simulink model "tx2"  (R2022a)
settings: Solver=FixedStepDiscrete  StartTime=0.0  StopTime=3.1e6  FixedStep=1  RelTol=1e-3
undefined symbols (not defined in the file or in its folder): rom_bf1, rom_bf2, rom_bf3, rom_bf4, rom_bf5, rom_bf6, rom_bf7, rom_bf8, rom_pilot_tt
libraries: hdlsllib x809, whdlutilities x460, whdlmod x104, whdledac x26, simulink x3
(part 4 of 27)

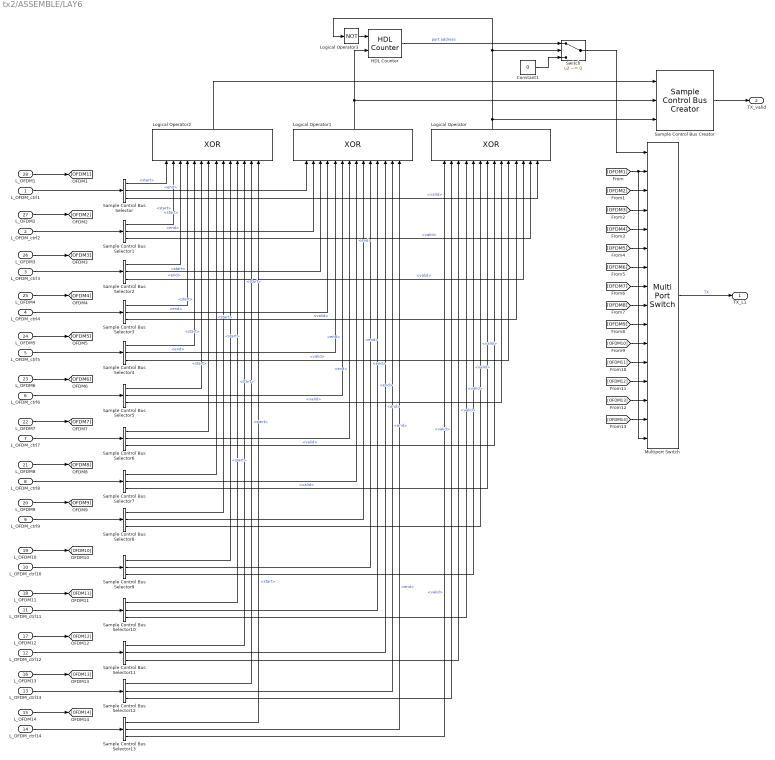
== system tx2/ASSEMBLE/LAY6 ==
  L_OFDM_ctrl1 : Inport  OutDataTypeStr=Bus: samplecontrol
  L_OFDM_ctrl2 : Inport  Port=2  OutDataTypeStr=Bus: samplecontrol
  L_OFDM_ctrl3 : Inport  Port=3  OutDataTypeStr=Bus: samplecontrol
  L_OFDM_ctrl4 : Inport  Port=4  OutDataTypeStr=Bus: samplecontrol
  L_OFDM_ctrl5 : Inport  Port=5  OutDataTypeStr=Bus: samplecontrol
  L_OFDM_ctrl6 : Inport  Port=6  OutDataTypeStr=Bus: samplecontrol
  L_OFDM_ctrl7 : Inport  Port=7  OutDataTypeStr=Bus: samplecontrol
  L_OFDM_ctrl8 : Inport  Port=8  OutDataTypeStr=Bus: samplecontrol
  L_OFDM_ctrl9 : Inport  Port=9  OutDataTypeStr=Bus: samplecontrol
  L_OFDM_ctrl10 : Inport  Port=10  OutDataTypeStr=Bus: samplecontrol
  L_OFDM_ctrl11 : Inport  Port=11  OutDataTypeStr=Bus: samplecontrol
  L_OFDM_ctrl12 : Inport  Port=12  OutDataTypeStr=Bus: samplecontrol
  L_OFDM_ctrl13 : Inport  Port=13  OutDataTypeStr=Bus: samplecontrol
  L_OFDM_ctrl14 : Inport  Port=14  OutDataTypeStr=Bus: samplecontrol
  L_OFDM14 : Inport  Port=15
  L_OFDM13 : Inport  Port=16
  L_OFDM12 : Inport  Port=17
  L_OFDM11 : Inport  Port=18
  L_OFDM10 : Inport  Port=19
  L_OFDM9 : Inport  Port=20
  L_OFDM8 : Inport  Port=21
  L_OFDM7 : Inport  Port=22
  L_OFDM6 : Inport  Port=23
  L_OFDM5 : Inport  Port=24
  L_OFDM4 : Inport  Port=25
  L_OFDM3 : Inport  Port=26
  L_OFDM2 : Inport  Port=27
  L_OFDM1 : Inport  Port=28
  Constant1 : Constant  Value=0  OutDataTypeStr=uint8
  HDL Counter : hdlsllib/Sources/HDL Counter  CountType=Count limited  CountInit=0  CountStep=1  CountMax=13  CountFromType=Initial value  CountFrom=0  CountResetPort=on  CountLoadPort=off  CountEnbPort=on  CountDirPort=off  CountHitOutputPort=off  CountDataType=Unsigned  CountWordLen=8  CountFracLen=0  CountSampTime=1
  Logical Operator : Logic  Operator=XOR  Inputs=14  AllPortsSameDT=off  OutDataTypeStr=boolean
  Logical Operator1 : Logic  Operator=XOR  Inputs=14  AllPortsSameDT=off  OutDataTypeStr=boolean
  Logical Operator2 : Logic  Operator=XOR  Inputs=14  AllPortsSameDT=off  OutDataTypeStr=boolean
  Logical Operator3 : Logic  Operator=NOT  AllPortsSameDT=off  OutDataTypeStr=boolean
  Multiport Switch : MultiPortSwitch  DataPortOrder=Zero-based contiguous  Inputs=14  DataPortForDefault=Additional data port  zeroidx=on  SaturateOnIntegerOverflow=off  InputSameDT=off
  Sample Control Bus Creator : whdlutilities/Sample Control Bus Creator
      settings: SourceProductBaseCode=LH
  Sample Control Bus Selector{,1..13} (14 alike) : whdlutilities/Sample Control Bus Selector  OutputSignals=start,end,valid
      settings: SourceProductBaseCode=LH
  Switch : Switch  Criteria=u2 ~= 0  SaturateOnIntegerOverflow=off  InputSameDT=off
  TX_L1 : Outport
  TX_valid : Outport  Port=2  OutDataTypeStr=Bus: samplecontrol
  wires:
  Logical Operator2/1 -> Sample Control Bus Creator/1
  Sample Control Bus Creator/1 -> TX_valid/1
  Sample Control Bus Selector13/1 -> Logical Operator2/14  "<start>"
  Sample Control Bus Selector12/1 -> Logical Operator2/13  "<start>"
  Sample Control Bus Selector11/1 -> Logical Operator2/12  "<start>"
  Sample Control Bus Selector10/1 -> Logical Operator2/11  "<start>"
  Sample Control Bus Selector9/1 -> Logical Operator2/10  "<start>"
  Sample Control Bus Selector8/1 -> Logical Operator2/9  "<start>"
  Sample Control Bus Selector7/1 -> Logical Operator2/8  "<start>"
  Sample Control Bus Selector6/1 -> Logical Operator2/7  "<start>"
  Sample Control Bus Selector5/1 -> Logical Operator2/6  "<start>"
  Sample Control Bus Selector4/1 -> Logical Operator2/5  "<start>"
  Sample Control Bus Selector3/1 -> Logical Operator2/4  "<start>"
  Sample Control Bus Selector2/1 -> Logical Operator2/3  "<start>"
  Sample Control Bus Selector1/1 -> Logical Operator2/2  "<start>"
  Sample Control Bus Selector/1 -> Logical Operator2/1  "<start>"
  Multiport Switch/1 -> TX_L1/1  "TX"
  L_OFDM_ctrl11/1 -> Sample Control Bus Selector10/1
  L_OFDM9/1 -> [OFDM9]
  L_OFDM_ctrl1/1 -> Sample Control Bus Selector/1
  L_OFDM_ctrl7/1 -> Sample Control Bus Selector6/1
  L_OFDM_ctrl4/1 -> Sample Control Bus Selector3/1
  L_OFDM_ctrl14/1 -> Sample Control Bus Selector13/1
  L_OFDM_ctrl9/1 -> Sample Control Bus Selector8/1
  L_OFDM_ctrl3/1 -> Sample Control Bus Selector2/1
  L_OFDM7/1 -> [OFDM7]
  L_OFDM6/1 -> [OFDM6]
  L_OFDM14/1 -> [OFDM14]
  L_OFDM_ctrl2/1 -> Sample Control Bus Selector1/1
  L_OFDM_ctrl13/1 -> Sample Control Bus Selector12/1
  Sample Control Bus Selector9/3 -> Logical Operator/5  "<valid>"
  Sample Control Bus Selector9/2 -> Logical Operator1/10  "<end>"
  L_OFDM_ctrl5/1 -> Sample Control Bus Selector4/1
  Sample Control Bus Selector7/2 -> Logical Operator1/8  "<end>"
  L_OFDM_ctrl12/1 -> Sample Control Bus Selector11/1
  [OFDM8] -> Multiport Switch/9
  Sample Control Bus Selector1/2 -> Logical Operator1/2  "<end>"
  Sample Control Bus Selector3/2 -> Logical Operator1/4  "<end>"
  Sample Control Bus Selector13/3 -> Logical Operator/1  "<valid>"
  Sample Control Bus Selector3/3 -> Logical Operator/11  "<valid>"
  [OFDM3] -> Multiport Switch/4
  Sample Control Bus Selector4/2 -> Logical Operator1/5  "<end>"
  Sample Control Bus Selector11/3 -> Logical Operator/3  "<valid>"
  [OFDM11] -> Multiport Switch/12
  L_OFDM4/1 -> [OFDM4]
  Sample Control Bus Selector11/2 -> Logical Operator1/12  "<end>"
  Sample Control Bus Selector4/3 -> Logical Operator/10  "<valid>"
  [OFDM12] -> Multiport Switch/13
  Sample Control Bus Selector2/2 -> Logical Operator1/3  "<end>"
  L_OFDM1/1 -> [OFDM1]
  Constant1/1 -> Switch/3
  L_OFDM11/1 -> [OFDM11]
  L_OFDM12/1 -> [OFDM12]
  Sample Control Bus Selector/2 -> Logical Operator1/1  "<end>"
  Sample Control Bus Selector5/3 -> Logical Operator/9  "<valid>"
  Switch/1 -> Multiport Switch/1
  Sample Control Bus Selector2/3 -> Logical Operator/12  "<valid>"
  [OFDM13] -> Multiport Switch/14
  [OFDM4] -> Multiport Switch/5
  [OFDM5] -> Multiport Switch/6
  HDL Counter/1 -> Switch/1  "port address"
  L_OFDM13/1 -> [OFDM13]
  [OFDM10] -> Multiport Switch/11
  Sample Control Bus Selector8/2 -> Logical Operator1/9  "<end>"
  Sample Control Bus Selector7/3 -> Logical Operator/7  "<valid>"
  L_OFDM_ctrl10/1 -> Sample Control Bus Selector9/1
  L_OFDM_ctrl6/1 -> Sample Control Bus Selector5/1
  [OFDM1] -> Multiport Switch/16, Multiport Switch/2
  Sample Control Bus Selector12/2 -> Logical Operator1/13  "<end>"
  Sample Control Bus Selector13/2 -> Logical Operator1/14  "<end>"
  L_OFDM10/1 -> [OFDM10]
  Sample Control Bus Selector6/2 -> Logical Operator1/7  "<end>"
  [OFDM7] -> Multiport Switch/8
  [OFDM6] -> Multiport Switch/7
  Logical Operator/1 -> Sample Control Bus Creator/3, Switch/2, Logical Operator3/1
  Sample Control Bus Selector6/3 -> Logical Operator/8  "<valid>"
  Sample Control Bus Selector5/2 -> Logical Operator1/6  "<end>"
  [OFDM9] -> Multiport Switch/10
  [OFDM2] -> Multiport Switch/3
  L_OFDM2/1 -> [OFDM2]
  Sample Control Bus Selector12/3 -> Logical Operator/2  "<valid>"
  L_OFDM3/1 -> [OFDM3]
  Sample Control Bus Selector1/3 -> Logical Operator/13  "<valid>"
  L_OFDM8/1 -> [OFDM8]
  Sample Control Bus Selector10/2 -> Logical Operator1/11  "<end>"
  Sample Control Bus Selector/3 -> Logical Operator/14  "<valid>"
  L_OFDM5/1 -> [OFDM5]
  Logical Operator1/1 -> Sample Control Bus Creator/2, HDL Counter/2
  [OFDM14] -> Multiport Switch/15
  Sample Control Bus Selector10/3 -> Logical Operator/4  "<valid>"
  L_OFDM_ctrl8/1 -> Sample Control Bus Selector7/1
  Sample Control Bus Selector8/3 -> Logical Operator/6  "<valid>"
  Logical Operator3/1 -> HDL Counter/1

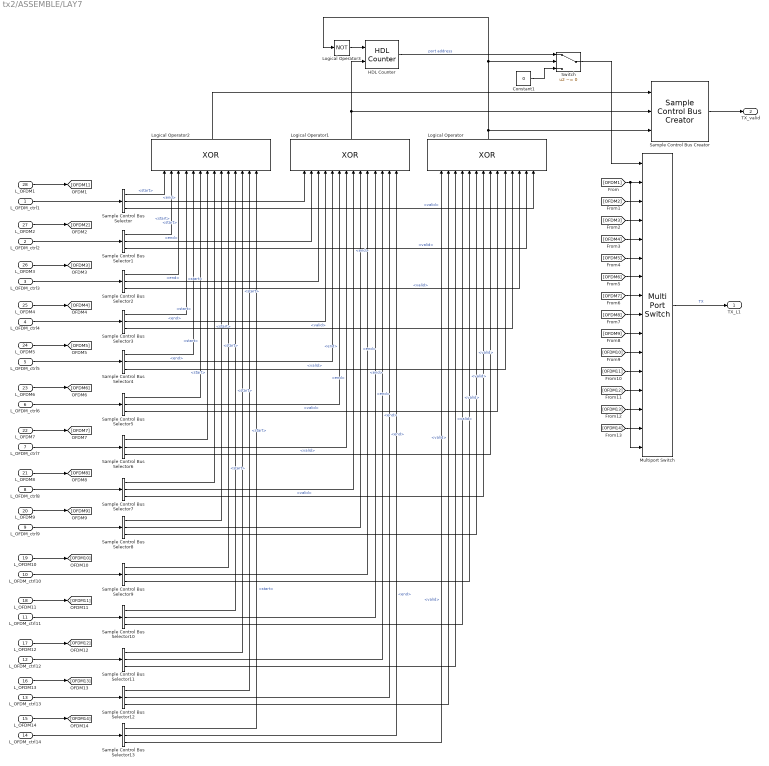
== system tx2/ASSEMBLE/LAY7 ==
  L_OFDM_ctrl1 : Inport  OutDataTypeStr=Bus: samplecontrol
  L_OFDM_ctrl2 : Inport  Port=2  OutDataTypeStr=Bus: samplecontrol
  L_OFDM_ctrl3 : Inport  Port=3  OutDataTypeStr=Bus: samplecontrol
  L_OFDM_ctrl4 : Inport  Port=4  OutDataTypeStr=Bus: samplecontrol
  L_OFDM_ctrl5 : Inport  Port=5  OutDataTypeStr=Bus: samplecontrol
  L_OFDM_ctrl6 : Inport  Port=6  OutDataTypeStr=Bus: samplecontrol
  L_OFDM_ctrl7 : Inport  Port=7  OutDataTypeStr=Bus: samplecontrol
  L_OFDM_ctrl8 : Inport  Port=8  OutDataTypeStr=Bus: samplecontrol
  L_OFDM_ctrl9 : Inport  Port=9  OutDataTypeStr=Bus: samplecontrol
  L_OFDM_ctrl10 : Inport  Port=10  OutDataTypeStr=Bus: samplecontrol
  L_OFDM_ctrl11 : Inport  Port=11  OutDataTypeStr=Bus: samplecontrol
  L_OFDM_ctrl12 : Inport  Port=12  OutDataTypeStr=Bus: samplecontrol
  L_OFDM_ctrl13 : Inport  Port=13  OutDataTypeStr=Bus: samplecontrol
  L_OFDM_ctrl14 : Inport  Port=14  OutDataTypeStr=Bus: samplecontrol
  L_OFDM14 : Inport  Port=15
  L_OFDM13 : Inport  Port=16
  L_OFDM12 : Inport  Port=17
  L_OFDM11 : Inport  Port=18
  L_OFDM10 : Inport  Port=19
  L_OFDM9 : Inport  Port=20
  L_OFDM8 : Inport  Port=21
  L_OFDM7 : Inport  Port=22
  L_OFDM6 : Inport  Port=23
  L_OFDM5 : Inport  Port=24
  L_OFDM4 : Inport  Port=25
  L_OFDM3 : Inport  Port=26
  L_OFDM2 : Inport  Port=27
  L_OFDM1 : Inport  Port=28
  Constant1 : Constant  Value=0  OutDataTypeStr=uint8
  HDL Counter : hdlsllib/Sources/HDL Counter  CountType=Count limited  CountInit=0  CountStep=1  CountMax=13  CountFromType=Initial value  CountFrom=0  CountResetPort=on  CountLoadPort=off  CountEnbPort=on  CountDirPort=off  CountHitOutputPort=off  CountDataType=Unsigned  CountWordLen=8  CountFracLen=0  CountSampTime=1
  Logical Operator : Logic  Operator=XOR  Inputs=14  AllPortsSameDT=off  OutDataTypeStr=boolean
  Logical Operator1 : Logic  Operator=XOR  Inputs=14  AllPortsSameDT=off  OutDataTypeStr=boolean
  Logical Operator2 : Logic  Operator=XOR  Inputs=14  AllPortsSameDT=off  OutDataTypeStr=boolean
  Logical Operator3 : Logic  Operator=NOT  AllPortsSameDT=off  OutDataTypeStr=boolean
  Multiport Switch : MultiPortSwitch  DataPortOrder=Zero-based contiguous  Inputs=14  DataPortForDefault=Additional data port  zeroidx=on  SaturateOnIntegerOverflow=off  InputSameDT=off
  Sample Control Bus Creator : whdlutilities/Sample Control Bus Creator
      settings: SourceProductBaseCode=LH
  Sample Control Bus Selector{,1..13} (14 alike) : whdlutilities/Sample Control Bus Selector  OutputSignals=start,end,valid
      settings: SourceProductBaseCode=LH
  Switch : Switch  Criteria=u2 ~= 0  SaturateOnIntegerOverflow=off  InputSameDT=off
  TX_L1 : Outport
  TX_valid : Outport  Port=2  OutDataTypeStr=Bus: samplecontrol
  wires:
  Sample Control Bus Selector8/3 -> Logical Operator/6  "<valid>"
  L_OFDM_ctrl8/1 -> Sample Control Bus Selector7/1
  Sample Control Bus Selector10/3 -> Logical Operator/4  "<valid>"
  [OFDM14] -> Multiport Switch/15
  Logical Operator1/1 -> HDL Counter/2, Sample Control Bus Creator/2
  L_OFDM5/1 -> [OFDM5]
  Sample Control Bus Selector/3 -> Logical Operator/14  "<valid>"
  Sample Control Bus Selector10/2 -> Logical Operator1/11  "<end>"
  L_OFDM8/1 -> [OFDM8]
  Sample Control Bus Selector1/3 -> Logical Operator/13  "<valid>"
  L_OFDM3/1 -> [OFDM3]
  Sample Control Bus Selector12/3 -> Logical Operator/2  "<valid>"
  L_OFDM2/1 -> [OFDM2]
  [OFDM2] -> Multiport Switch/3
  [OFDM9] -> Multiport Switch/10
  Sample Control Bus Selector5/2 -> Logical Operator1/6  "<end>"
  Sample Control Bus Selector6/3 -> Logical Operator/8  "<valid>"
  Logical Operator/1 -> Switch/2, Logical Operator3/1, Sample Control Bus Creator/3
  [OFDM6] -> Multiport Switch/7
  [OFDM7] -> Multiport Switch/8
  Sample Control Bus Selector6/2 -> Logical Operator1/7  "<end>"
  L_OFDM10/1 -> [OFDM10]
  Sample Control Bus Selector13/2 -> Logical Operator1/14  "<end>"
  Sample Control Bus Selector12/2 -> Logical Operator1/13  "<end>"
  [OFDM1] -> Multiport Switch/16, Multiport Switch/2
  L_OFDM_ctrl6/1 -> Sample Control Bus Selector5/1
  L_OFDM_ctrl10/1 -> Sample Control Bus Selector9/1
  Sample Control Bus Selector7/3 -> Logical Operator/7  "<valid>"
  Sample Control Bus Selector8/2 -> Logical Operator1/9  "<end>"
  [OFDM10] -> Multiport Switch/11
  L_OFDM13/1 -> [OFDM13]
  HDL Counter/1 -> Switch/1  "port address"
  [OFDM5] -> Multiport Switch/6
  [OFDM4] -> Multiport Switch/5
  [OFDM13] -> Multiport Switch/14
  Sample Control Bus Selector2/3 -> Logical Operator/12  "<valid>"
  Switch/1 -> Multiport Switch/1
  Sample Control Bus Selector5/3 -> Logical Operator/9  "<valid>"
  Sample Control Bus Selector/2 -> Logical Operator1/1  "<end>"
  L_OFDM12/1 -> [OFDM12]
  L_OFDM11/1 -> [OFDM11]
  Constant1/1 -> Switch/3
  L_OFDM1/1 -> [OFDM1]
  Sample Control Bus Selector2/2 -> Logical Operator1/3  "<end>"
  [OFDM12] -> Multiport Switch/13
  Sample Control Bus Selector4/3 -> Logical Operator/10  "<valid>"
  Sample Control Bus Selector11/2 -> Logical Operator1/12  "<end>"
  L_OFDM4/1 -> [OFDM4]
  [OFDM11] -> Multiport Switch/12
  Sample Control Bus Selector11/3 -> Logical Operator/3  "<valid>"
  Sample Control Bus Selector4/2 -> Logical Operator1/5  "<end>"
  [OFDM3] -> Multiport Switch/4
  Sample Control Bus Selector3/3 -> Logical Operator/11  "<valid>"
  Sample Control Bus Selector13/3 -> Logical Operator/1  "<valid>"
  Sample Control Bus Selector3/2 -> Logical Operator1/4  "<end>"
  Sample Control Bus Selector1/2 -> Logical Operator1/2  "<end>"
  [OFDM8] -> Multiport Switch/9
  L_OFDM_ctrl12/1 -> Sample Control Bus Selector11/1
  Sample Control Bus Selector7/2 -> Logical Operator1/8  "<end>"
  L_OFDM_ctrl5/1 -> Sample Control Bus Selector4/1
  Sample Control Bus Selector9/2 -> Logical Operator1/10  "<end>"
  Sample Control Bus Selector9/3 -> Logical Operator/5  "<valid>"
  L_OFDM_ctrl13/1 -> Sample Control Bus Selector12/1
  L_OFDM_ctrl2/1 -> Sample Control Bus Selector1/1
  L_OFDM14/1 -> [OFDM14]
  L_OFDM6/1 -> [OFDM6]
  L_OFDM7/1 -> [OFDM7]
  L_OFDM_ctrl3/1 -> Sample Control Bus Selector2/1
  L_OFDM_ctrl9/1 -> Sample Control Bus Selector8/1
  L_OFDM_ctrl14/1 -> Sample Control Bus Selector13/1
  L_OFDM_ctrl4/1 -> Sample Control Bus Selector3/1
  L_OFDM_ctrl7/1 -> Sample Control Bus Selector6/1
  L_OFDM_ctrl1/1 -> Sample Control Bus Selector/1
  L_OFDM9/1 -> [OFDM9]
  L_OFDM_ctrl11/1 -> Sample Control Bus Selector10/1
  Multiport Switch/1 -> TX_L1/1  "TX"
  Sample Control Bus Selector/1 -> Logical Operator2/1  "<start>"
  Sample Control Bus Selector1/1 -> Logical Operator2/2  "<start>"
  Sample Control Bus Selector2/1 -> Logical Operator2/3  "<start>"
  Sample Control Bus Selector3/1 -> Logical Operator2/4  "<start>"
  Sample Control Bus Selector4/1 -> Logical Operator2/5  "<start>"
  Sample Control Bus Selector5/1 -> Logical Operator2/6  "<start>"
  Sample Control Bus Selector6/1 -> Logical Operator2/7  "<start>"
  Sample Control Bus Selector7/1 -> Logical Operator2/8  "<start>"
  Sample Control Bus Selector8/1 -> Logical Operator2/9  "<start>"
  Sample Control Bus Selector9/1 -> Logical Operator2/10  "<start>"
  Sample Control Bus Selector10/1 -> Logical Operator2/11  "<start>"
  Sample Control Bus Selector11/1 -> Logical Operator2/12  "<start>"
  Sample Control Bus Selector12/1 -> Logical Operator2/13  "<start>"
  Sample Control Bus Selector13/1 -> Logical Operator2/14  "<start>"
  Sample Control Bus Creator/1 -> TX_valid/1
  Logical Operator2/1 -> Sample Control Bus Creator/1
  Logical Operator3/1 -> HDL Counter/1

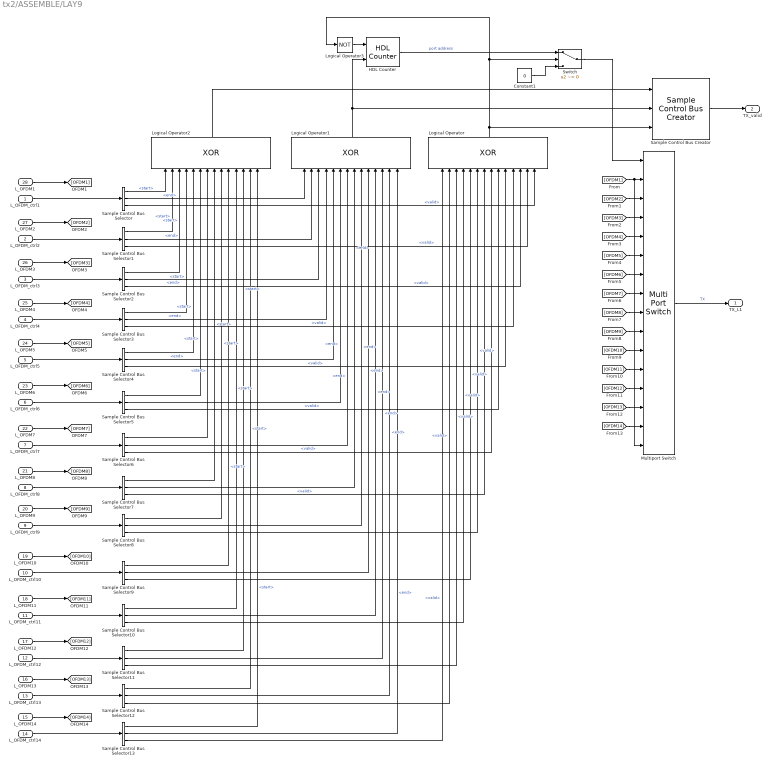
== system tx2/ASSEMBLE/LAY9 ==
  L_OFDM_ctrl1 : Inport  OutDataTypeStr=Bus: samplecontrol
  L_OFDM_ctrl2 : Inport  Port=2  OutDataTypeStr=Bus: samplecontrol
  L_OFDM_ctrl3 : Inport  Port=3  OutDataTypeStr=Bus: samplecontrol
  L_OFDM_ctrl4 : Inport  Port=4  OutDataTypeStr=Bus: samplecontrol
  L_OFDM_ctrl5 : Inport  Port=5  OutDataTypeStr=Bus: samplecontrol
  L_OFDM_ctrl6 : Inport  Port=6  OutDataTypeStr=Bus: samplecontrol
  L_OFDM_ctrl7 : Inport  Port=7  OutDataTypeStr=Bus: samplecontrol
  L_OFDM_ctrl8 : Inport  Port=8  OutDataTypeStr=Bus: samplecontrol
  L_OFDM_ctrl9 : Inport  Port=9  OutDataTypeStr=Bus: samplecontrol
  L_OFDM_ctrl10 : Inport  Port=10  OutDataTypeStr=Bus: samplecontrol
  L_OFDM_ctrl11 : Inport  Port=11  OutDataTypeStr=Bus: samplecontrol
  L_OFDM_ctrl12 : Inport  Port=12  OutDataTypeStr=Bus: samplecontrol
  L_OFDM_ctrl13 : Inport  Port=13  OutDataTypeStr=Bus: samplecontrol
  L_OFDM_ctrl14 : Inport  Port=14  OutDataTypeStr=Bus: samplecontrol
  L_OFDM14 : Inport  Port=15
  L_OFDM13 : Inport  Port=16
  L_OFDM12 : Inport  Port=17
  L_OFDM11 : Inport  Port=18
  L_OFDM10 : Inport  Port=19
  L_OFDM9 : Inport  Port=20
  L_OFDM8 : Inport  Port=21
  L_OFDM7 : Inport  Port=22
  L_OFDM6 : Inport  Port=23
  L_OFDM5 : Inport  Port=24
  L_OFDM4 : Inport  Port=25
  L_OFDM3 : Inport  Port=26
  L_OFDM2 : Inport  Port=27
  L_OFDM1 : Inport  Port=28
  Constant1 : Constant  Value=0  OutDataTypeStr=uint8
  HDL Counter : hdlsllib/Sources/HDL Counter  CountType=Count limited  CountInit=0  CountStep=1  CountMax=13  CountFromType=Initial value  CountFrom=0  CountResetPort=on  CountLoadPort=off  CountEnbPort=on  CountDirPort=off  CountHitOutputPort=off  CountDataType=Unsigned  CountWordLen=8  CountFracLen=0  CountSampTime=1
  Logical Operator : Logic  Operator=XOR  Inputs=14  AllPortsSameDT=off  OutDataTypeStr=boolean
  Logical Operator1 : Logic  Operator=XOR  Inputs=14  AllPortsSameDT=off  OutDataTypeStr=boolean
  Logical Operator2 : Logic  Operator=XOR  Inputs=14  AllPortsSameDT=off  OutDataTypeStr=boolean
  Logical Operator3 : Logic  Operator=NOT  AllPortsSameDT=off  OutDataTypeStr=boolean
  Multiport Switch : MultiPortSwitch  DataPortOrder=Zero-based contiguous  Inputs=14  DataPortForDefault=Additional data port  zeroidx=on  SaturateOnIntegerOverflow=off  InputSameDT=off
  Sample Control Bus Creator : whdlutilities/Sample Control Bus Creator
      settings: SourceProductBaseCode=LH
  Sample Control Bus Selector{,1..13} (14 alike) : whdlutilities/Sample Control Bus Selector  OutputSignals=start,end,valid
      settings: SourceProductBaseCode=LH
  Switch : Switch  Criteria=u2 ~= 0  SaturateOnIntegerOverflow=off  InputSameDT=off
  TX_L1 : Outport
  TX_valid : Outport  Port=2  OutDataTypeStr=Bus: samplecontrol
  wires:
  Logical Operator2/1 -> Sample Control Bus Creator/1
  Sample Control Bus Creator/1 -> TX_valid/1
  Sample Control Bus Selector13/1 -> Logical Operator2/14  "<start>"
  Sample Control Bus Selector12/1 -> Logical Operator2/13  "<start>"
  Sample Control Bus Selector11/1 -> Logical Operator2/12  "<start>"
  Sample Control Bus Selector10/1 -> Logical Operator2/11  "<start>"
  Sample Control Bus Selector9/1 -> Logical Operator2/10  "<start>"
  Sample Control Bus Selector8/1 -> Logical Operator2/9  "<start>"
  Sample Control Bus Selector7/1 -> Logical Operator2/8  "<start>"
  Sample Control Bus Selector6/1 -> Logical Operator2/7  "<start>"
  Sample Control Bus Selector5/1 -> Logical Operator2/6  "<start>"
  Sample Control Bus Selector4/1 -> Logical Operator2/5  "<start>"
  Sample Control Bus Selector3/1 -> Logical Operator2/4  "<start>"
  Sample Control Bus Selector2/1 -> Logical Operator2/3  "<start>"
  Sample Control Bus Selector1/1 -> Logical Operator2/2  "<start>"
  Sample Control Bus Selector/1 -> Logical Operator2/1  "<start>"
  Multiport Switch/1 -> TX_L1/1  "TX"
  L_OFDM_ctrl11/1 -> Sample Control Bus Selector10/1
  L_OFDM9/1 -> [OFDM9]
  L_OFDM_ctrl1/1 -> Sample Control Bus Selector/1
  L_OFDM_ctrl7/1 -> Sample Control Bus Selector6/1
  L_OFDM_ctrl4/1 -> Sample Control Bus Selector3/1
  L_OFDM_ctrl14/1 -> Sample Control Bus Selector13/1
  L_OFDM_ctrl9/1 -> Sample Control Bus Selector8/1
  L_OFDM_ctrl3/1 -> Sample Control Bus Selector2/1
  L_OFDM7/1 -> [OFDM7]
  L_OFDM6/1 -> [OFDM6]
  L_OFDM14/1 -> [OFDM14]
  L_OFDM_ctrl2/1 -> Sample Control Bus Selector1/1
  L_OFDM_ctrl13/1 -> Sample Control Bus Selector12/1
  Sample Control Bus Selector9/3 -> Logical Operator/5  "<valid>"
  Sample Control Bus Selector9/2 -> Logical Operator1/10  "<end>"
  L_OFDM_ctrl5/1 -> Sample Control Bus Selector4/1
  Sample Control Bus Selector7/2 -> Logical Operator1/8  "<end>"
  L_OFDM_ctrl12/1 -> Sample Control Bus Selector11/1
  [OFDM8] -> Multiport Switch/9
  Sample Control Bus Selector1/2 -> Logical Operator1/2  "<end>"
  Sample Control Bus Selector3/2 -> Logical Operator1/4  "<end>"
  Sample Control Bus Selector13/3 -> Logical Operator/1  "<valid>"
  Sample Control Bus Selector3/3 -> Logical Operator/11  "<valid>"
  [OFDM3] -> Multiport Switch/4
  Sample Control Bus Selector4/2 -> Logical Operator1/5  "<end>"
  Sample Control Bus Selector11/3 -> Logical Operator/3  "<valid>"
  [OFDM11] -> Multiport Switch/12
  L_OFDM4/1 -> [OFDM4]
  Sample Control Bus Selector11/2 -> Logical Operator1/12  "<end>"
  Sample Control Bus Selector4/3 -> Logical Operator/10  "<valid>"
  [OFDM12] -> Multiport Switch/13
  Sample Control Bus Selector2/2 -> Logical Operator1/3  "<end>"
  L_OFDM1/1 -> [OFDM1]
  Constant1/1 -> Switch/3
  L_OFDM11/1 -> [OFDM11]
  L_OFDM12/1 -> [OFDM12]
  Sample Control Bus Selector/2 -> Logical Operator1/1  "<end>"
  Sample Control Bus Selector5/3 -> Logical Operator/9  "<valid>"
  Switch/1 -> Multiport Switch/1
  Sample Control Bus Selector2/3 -> Logical Operator/12  "<valid>"
  [OFDM13] -> Multiport Switch/14
  [OFDM4] -> Multiport Switch/5
  [OFDM5] -> Multiport Switch/6
  HDL Counter/1 -> Switch/1  "port address"
  L_OFDM13/1 -> [OFDM13]
  [OFDM10] -> Multiport Switch/11
  Sample Control Bus Selector8/2 -> Logical Operator1/9  "<end>"
  Sample Control Bus Selector7/3 -> Logical Operator/7  "<valid>"
  L_OFDM_ctrl10/1 -> Sample Control Bus Selector9/1
  L_OFDM_ctrl6/1 -> Sample Control Bus Selector5/1
  [OFDM1] -> Multiport Switch/16, Multiport Switch/2
  Sample Control Bus Selector12/2 -> Logical Operator1/13  "<end>"
  Sample Control Bus Selector13/2 -> Logical Operator1/14  "<end>"
  L_OFDM10/1 -> [OFDM10]
  Sample Control Bus Selector6/2 -> Logical Operator1/7  "<end>"
  [OFDM7] -> Multiport Switch/8
  [OFDM6] -> Multiport Switch/7
  Logical Operator/1 -> Sample Control Bus Creator/3, Switch/2, Logical Operator3/1
  Sample Control Bus Selector6/3 -> Logical Operator/8  "<valid>"
  Sample Control Bus Selector5/2 -> Logical Operator1/6  "<end>"
  [OFDM9] -> Multiport Switch/10
  [OFDM2] -> Multiport Switch/3
  L_OFDM2/1 -> [OFDM2]
  Sample Control Bus Selector12/3 -> Logical Operator/2  "<valid>"
  L_OFDM3/1 -> [OFDM3]
  Sample Control Bus Selector1/3 -> Logical Operator/13  "<valid>"
  L_OFDM8/1 -> [OFDM8]
  Sample Control Bus Selector10/2 -> Logical Operator1/11  "<end>"
  Sample Control Bus Selector/3 -> Logical Operator/14  "<valid>"
  L_OFDM5/1 -> [OFDM5]
  Logical Operator1/1 -> Sample Control Bus Creator/2, HDL Counter/2
  [OFDM14] -> Multiport Switch/15
  Sample Control Bus Selector10/3 -> Logical Operator/4  "<valid>"
  L_OFDM_ctrl8/1 -> Sample Control Bus Selector7/1
  Sample Control Bus Selector8/3 -> Logical Operator/6  "<valid>"
  Logical Operator3/1 -> HDL Counter/1

== system tx2/NR DL process0/Subsystem1 ==
  start : Inport
  Compare To Constant : simulink/Logic and Bit Operations/Compare To Constant  relop===  const=valid_length  OutDataTypeStr=boolean
  Data Type Conversion : DataTypeConversion  OutDataTypeStr=boolean  SaturateOnIntegerOverflow=off  RndMeth=Floor
  Delay2 : Delay  DelayLength=1  InitialCondition=0
  HDL Counter1 : hdlsllib/Sources/HDL Counter  CountType=Count limited  CountInit=1  CountStep=1  CountMax=valid_length  CountFromType=Initial value  CountFrom=1  CountResetPort=off  CountLoadPort=off  CountEnbPort=on  CountDirPort=off  CountHitOutputPort=off  CountDataType=Unsigned  CountWordLen=16  CountFracLen=0  CountSampTime=1
  HDL Counter4 : hdlsllib/Sources/HDL Counter  CountType=Count limited  CountInit=0  CountStep=1  CountMax=1  CountFromType=Initial value  CountFrom=0  CountResetPort=on  CountLoadPort=off  CountEnbPort=on  CountDirPort=off  CountHitOutputPort=off  CountDataType=Unsigned  CountWordLen=8  CountFracLen=0  CountSampTime=1
  valid_out : Outport
  wires:
  Compare To Constant/1 -> HDL Counter4/1
  HDL Counter1/1 -> Compare To Constant/1  "count_1"
  HDL Counter4/1 -> Data Type Conversion/1
  start/1 -> HDL Counter4/2
  Data Type Conversion/1 -> Delay2/1, HDL Counter1/1
  Delay2/1 -> valid_out/1  "valid_out"

== system tx2/NR DL process0/Subsystem2 ==
  start : Inport
  Compare To Constant : simulink/Logic and Bit Operations/Compare To Constant  relop===  const=valid_length  OutDataTypeStr=boolean
  Data Type Conversion : DataTypeConversion  OutDataTypeStr=boolean  SaturateOnIntegerOverflow=off  RndMeth=Floor
  Delay1 : Delay  InitialCondition=0
  Delay2 : Delay  DelayLength=1  InitialCondition=0
  Detect Fall Nonpositive : simulink/Logic and Bit Operations/Detect Fall Nonpositive  vinit=0  OutDataTypeStr=boolean
      settings: SourceProductBaseCode=SL
  HDL Counter1 : hdlsllib/Sources/HDL Counter  CountType=Count limited  CountInit=1  CountStep=1  CountMax=valid_length  CountFromType=Initial value  CountFrom=1  CountResetPort=off  CountLoadPort=off  CountEnbPort=on  CountDirPort=off  CountHitOutputPort=off  CountDataType=Unsigned  CountWordLen=16  CountFracLen=0  CountSampTime=1
  HDL Counter4 : hdlsllib/Sources/HDL Counter  CountType=Count limited  CountInit=0  CountStep=1  CountMax=1  CountFromType=Initial value  CountFrom=0  CountResetPort=on  CountLoadPort=off  CountEnbPort=on  CountDirPort=off  CountHitOutputPort=off  CountDataType=Unsigned  CountWordLen=8  CountFracLen=0  CountSampTime=1
  Logical Operator4 : Logic  AllPortsSameDT=off  OutDataTypeStr=boolean
  valid_out : Outport
  start_out : Outport  Port=2
  end_out : Outport  Port=3
  wires:
  Compare To Constant/1 -> HDL Counter4/1
  HDL Counter1/1 -> Compare To Constant/1  "count_1"
  HDL Counter4/1 -> Data Type Conversion/1
  start/1 -> Delay1/1, HDL Counter4/2
  Detect Fall Nonpositive/1 -> Logical Operator4/1  "symbol_end"
  Data Type Conversion/1 -> Delay2/1, Detect Fall Nonpositive/1, HDL Counter1/1
  Delay1/1 -> start_out/1  "start_out"
  Delay2/1 -> Logical Operator4/2, valid_out/1  "valid_out"
  Logical Operator4/1 -> end_out/1  "end_out"

== system tx2/NR DL process0/rom_bf2 ==
  note: HDL ROM
  note: rom_pilot = [1+1j;0+0j;-1+1j;0+0j;-1-1j;0+0j;1-1j;0+0j]*1/sqrt(2);
      | rom_pilot = repmat(rom_pilot,792/8,1);
      | rom_pilot = [rom_pilot;zeros(1024-792,1)];
      | rom_pilot_ofdm = ofdmmod(rom_pilot,1024,136);
      | rom_pilot_tt = fi(rom_pilot_ofdm,1,16,14);
  address : Inport
  Direct Lookup Table (n-D) : LookupNDDirect  NumberOfTableDimensions=1  Table=rom_pilot_tt  DiagnosticForOutOfRangeInput=Error
  InputReg : Delay  DelayLength=1
  ResetNoneDelay : Delay  DelayLength=1
  data_out : Outport
  wires:
  ResetNoneDelay/1 -> data_out/1
  address/1 -> InputReg/1
  Direct Lookup Table (n-D)/1 -> ResetNoneDelay/1
  InputReg/1 -> Direct Lookup Table (n-D)/1  "rom_add"

== system tx2/Subsystem1/BF ==
  layer_data_in1 : Inport
  BF_data_ctrl : Inport  Port=2  OutDataTypeStr=Bus: samplecontrol
  RB_id : Inport  Port=3  OutDataTypeStr=uint8
  RB_id_ctrl : Inport  Port=4  OutDataTypeStr=Bus: samplecontrol
  Delay{,3..8,10} (8 alike) : Delay  DelayLength=1  InitialCondition=0
  Delay1 : Delay  InitialCondition=0
  Delay2 : Delay  DelayLength=3  InitialCondition=0
  Delay9 : Delay  InitialCondition=0
  Logical Operator : Logic  Operator=NOT  AllPortsSameDT=off  OutDataTypeStr=boolean
  Mux : Mux  Inputs=8
  Product{,1..7} (8 alike) : Product  OutDataTypeStr=fixdt(1,16,14)  LockScale=on
  Sample Control Bus Selector : whdlutilities/Sample Control Bus Selector  OutputSignals=start,end,valid
      settings: SourceProductBaseCode=LH
  Sample Control Bus Selector1 : whdlutilities/Sample Control Bus Selector  OutputSignals=start,end,valid
      settings: SourceProductBaseCode=LH
  address controller : hdlsllib/Sources/HDL Counter  CountType=Count limited  CountInit=0  CountStep=1  CountMax=7  CountFromType=Initial value  CountFrom=0  CountResetPort=on  CountLoadPort=off  CountEnbPort=on  CountDirPort=off  CountHitOutputPort=off  CountDataType=Unsigned  CountWordLen=8  CountFracLen=0  CountSampTime=1
  rom_bf1 : Subsystem
  rom_bf2 : Subsystem
  rom_bf3 : Subsystem
  rom_bf4 : Subsystem
  rom_bf5 : Subsystem
  rom_bf6 : Subsystem
  rom_bf7 : Subsystem
  rom_bf8 : Subsystem
  process_bf : Outport  PortDimensions=8  VectorParamsAs1DForOutWhenUnconnected=off
  BF_ctrl : Outport  Port=2  OutDataTypeStr=Bus: samplecontrol  VectorParamsAs1DForOutWhenUnconnected=off
  RB_n_bf : Outport  Port=3  VectorParamsAs1DForOutWhenUnconnected=off
  wires:
  Delay1/1 -> Product7/1, Product6/1, Product5/1, Product4/1, Product3/1, Product2/1, Product1/1, Product/1
  rom_bf1/1(data_out) -> Product/2
  Product/1 -> Delay/1
  Delay2/1 -> BF_ctrl/1  "BF_ctrl"
  address controller/1 -> rom_bf7/1(address), rom_bf8/1(address), rom_bf6/1(address), rom_bf5/1(address), rom_bf4/1(address), rom_bf3/1(address), rom_bf2/1(address), rom_bf1/1(address)
  Delay9/1 -> RB_n_bf/1  "RB_ID"
  RB_id_ctrl/1 -> Sample Control Bus Selector1/1
  BF_data_ctrl/1 -> Delay2/1, Sample Control Bus Selector/1
  Sample Control Bus Selector1/2 -> address controller/2  "<end>"
  RB_id/1 -> Delay9/1
  layer_data_in1/1 -> Delay1/1
  Sample Control Bus Selector/3 -> rom_bf2/2(read_en), rom_bf1/2(read_en), rom_bf3/2(read_en), rom_bf4/2(read_en), rom_bf5/2(read_en), rom_bf6/2(read_en), rom_bf7/2(read_en), rom_bf8/2(read_en)  "<valid>"
  Product1/1 -> Delay3/1
  Product2/1 -> Delay4/1
  Product4/1 -> Delay6/1
  Product3/1 -> Delay5/1
  Product5/1 -> Delay7/1
  Product6/1 -> Delay8/1
  rom_bf2/1(data_out) -> Product1/2
  rom_bf3/1(data_out) -> Product2/2
  rom_bf4/1(data_out) -> Product3/2
  rom_bf5/1(data_out) -> Product4/2
  rom_bf6/1(data_out) -> Product5/2
  Product7/1 -> Delay10/1
  rom_bf7/1(data_out) -> Product6/2
  rom_bf8/1(data_out) -> Product7/2
  Delay3/1 -> Mux/2
  Delay4/1 -> Mux/3
  Delay5/1 -> Mux/4
  Delay10/1 -> Mux/8
  Delay8/1 -> Mux/7
  Delay7/1 -> Mux/6
  Delay6/1 -> Mux/5
  Delay/1 -> Mux/1
  Mux/1 -> process_bf/1
  Sample Control Bus Selector1/3 -> Logical Operator/1  "<valid>"
  Logical Operator/1 -> address controller/1

== system tx2/Subsystem1/OFDM_process1 ==
  process_bf : Inport
  BF_ctrl : Inport  Port=2
  Demux : Demux  Outputs=8
  OFDM_process1_bf1 : Subsystem
  OFDM_process1_bf2 : Subsystem
  OFDM_process1_bf3 : Subsystem
  OFDM_process1_bf4 : Subsystem
  OFDM_process1_bf5 : Subsystem
  OFDM_process1_bf6 : Subsystem
  OFDM_process1_bf7 : Subsystem
  OFDM_process1_bf8 : Subsystem
  OFDM_bf1 : Outport
  OFDM_ctrl_bf1 : Outport  Port=2
  OFDM_bf2 : Outport  Port=3
  OFDM_ctrl_bf2 : Outport  Port=4
  OFDM_bf3 : Outport  Port=5
  OFDM_ctrl_bf3 : Outport  Port=6
  OFDM_bf4 : Outport  Port=7
  OFDM_ctrl_bf4 : Outport  Port=8
  OFDM_bf5 : Outport  Port=9
  OFDM_ctrl_bf5 : Outport  Port=10
  OFDM_bf6 : Outport  Port=11
  OFDM_ctrl_bf6 : Outport  Port=12
  OFDM_bf7 : Outport  Port=13
  OFDM_ctrl_bf7 : Outport  Port=14
  OFDM_bf8 : Outport  Port=15
  OFDM_ctrl_bf8 : Outport  Port=16
  wires:
  Demux/3 -> OFDM_process1_bf3/1(data)  "bf3"
  Demux/1 -> OFDM_process1_bf1/1(data)  "bf1"
  BF_ctrl/1 -> OFDM_process1_bf7/2(BF_ctrl), OFDM_process1_bf8/2(BF_ctrl), OFDM_process1_bf6/2(BF_ctrl), OFDM_process1_bf5/2(BF_ctrl), OFDM_process1_bf4/2(BF_ctrl), OFDM_process1_bf3/2(BF_ctrl), OFDM_process1_bf2/2(BF_ctrl), OFDM_process1_bf1/2(BF_ctrl)
  Demux/5 -> OFDM_process1_bf5/1(data)  "bf5"
  OFDM_process1_bf1/2(OFDM_ctrl_process) -> OFDM_ctrl_bf1/1
  OFDM_process1_bf2/2(OFDM_ctrl_process) -> OFDM_ctrl_bf2/1
  Demux/2 -> OFDM_process1_bf2/1(data)  "bf2"
  Demux/4 -> OFDM_process1_bf4/1(data)  "bf4"
  OFDM_process1_bf8/2(OFDM_ctrl_process) -> OFDM_ctrl_bf8/1
  Demux/8 -> OFDM_process1_bf8/1(data)  "bf8"
  Demux/7 -> OFDM_process1_bf7/1(data)  "bf7"
  Demux/6 -> OFDM_process1_bf6/1(data)  "bf6"
  OFDM_process1_bf7/2(OFDM_ctrl_process) -> OFDM_ctrl_bf7/1
  OFDM_process1_bf6/1(OFDM_process) -> OFDM_bf6/1
  OFDM_process1_bf3/1(OFDM_process) -> OFDM_bf3/1
  OFDM_process1_bf6/2(OFDM_ctrl_process) -> OFDM_ctrl_bf6/1
  OFDM_process1_bf5/1(OFDM_process) -> OFDM_bf5/1
  OFDM_process1_bf1/1(OFDM_process) -> OFDM_bf1/1
  OFDM_process1_bf8/1(OFDM_process) -> OFDM_bf8/1
  OFDM_process1_bf4/2(OFDM_ctrl_process) -> OFDM_ctrl_bf4/1
  OFDM_process1_bf3/2(OFDM_ctrl_process) -> OFDM_ctrl_bf3/1
  OFDM_process1_bf5/2(OFDM_ctrl_process) -> OFDM_ctrl_bf5/1
  process_bf/1 -> Demux/1
  OFDM_process1_bf7/1(OFDM_process) -> OFDM_bf7/1
  OFDM_process1_bf4/1(OFDM_process) -> OFDM_bf4/1
  OFDM_process1_bf2/1(OFDM_process) -> OFDM_bf2/1

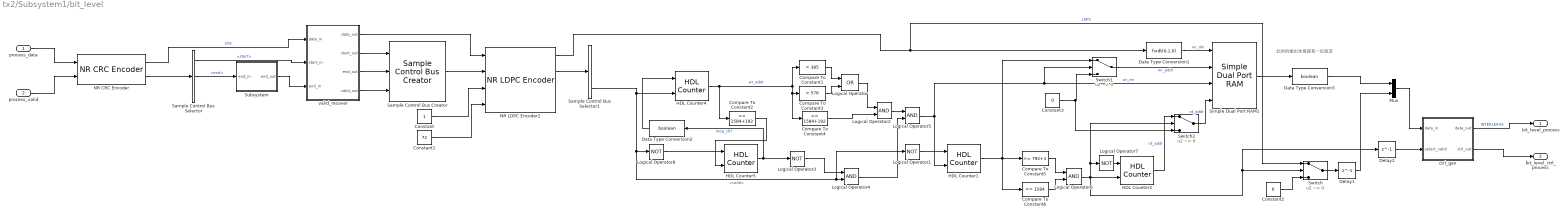
== system tx2/Subsystem1/bit_level ==
  note: 此时的输出本身具有一位延迟
  process_data : Inport
  process_valid : Inport  Port=2  OutDataTypeStr=Bus: samplecontrol
  Compare To Constant1 : hdlsllib/Logic and Bit Operations/Compare To Constant  relop=<  const=385  OutDataTypeStr=boolean
      settings: SourceProductBaseCode=SL
  Compare To Constant2 : hdlsllib/Logic and Bit Operations/Compare To Constant  relop===  const=1584+192  OutDataTypeStr=boolean
      settings: SourceProductBaseCode=SL
  Compare To Constant3 : hdlsllib/Logic and Bit Operations/Compare To Constant  relop=>  const=576  OutDataTypeStr=boolean
      settings: SourceProductBaseCode=SL
  Compare To Constant4 : hdlsllib/Logic and Bit Operations/Compare To Constant  relop=<=  const=1584+192  OutDataTypeStr=boolean
      settings: SourceProductBaseCode=SL
  Compare To Constant5 : hdlsllib/Logic and Bit Operations/Compare To Constant  relop=>=  const=792+1  OutDataTypeStr=boolean
      settings: SourceProductBaseCode=SL
  Compare To Constant6 : hdlsllib/Logic and Bit Operations/Compare To Constant  relop=<=  const=1584  OutDataTypeStr=boolean
      settings: SourceProductBaseCode=SL
  Constant : Constant  OutDataTypeStr=boolean
  Constant1 : Constant  Value=72  OutDataTypeStr=uint16
  Constant2 : Constant  Value=0  OutDataTypeStr=boolean
  Constant3 : Constant  Value=0  OutDataTypeStr=fixdt(0,12,0)
  Data Type Conversion1 : DataTypeConversion  OutDataTypeStr=fixdt(0,1,0)  SaturateOnIntegerOverflow=off  RndMeth=Floor
  Data Type Conversion2 : DataTypeConversion  OutDataTypeStr=boolean  SaturateOnIntegerOverflow=off  RndMeth=Floor
  Data Type Conversion3 : DataTypeConversion  OutDataTypeStr=boolean  SaturateOnIntegerOverflow=off  RndMeth=Floor
  Delay1 : Delay  DelayLength=1  InitialCondition=0
  Delay2 : Delay  DelayLength=1  InitialCondition=0
  HDL Counter1 : hdlsllib/Sources/HDL Counter  CountType=Count limited  CountInit=1  CountStep=1  CountMax=1584  CountFromType=Initial value  CountFrom=1  CountResetPort=on  CountLoadPort=off  CountEnbPort=on  CountDirPort=off  CountHitOutputPort=off  CountDataType=Unsigned  CountWordLen=12  CountFracLen=0  CountSampTime=1
  HDL Counter2 : hdlsllib/Sources/HDL Counter  CountType=Count limited  CountInit=1  CountStep=1  CountMax=792  CountFromType=Initial value  CountFrom=1  CountResetPort=on  CountLoadPort=off  CountEnbPort=on  CountDirPort=off  CountHitOutputPort=off  CountDataType=Unsigned  CountWordLen=12  CountFracLen=0  CountSampTime=1
  HDL Counter4 : hdlsllib/Sources/HDL Counter  CountType=Count limited  CountInit=1  CountStep=1  CountMax=4096-1  CountFromType=Initial value  CountFrom=1  CountResetPort=on  CountLoadPort=off  CountEnbPort=on  CountDirPort=off  CountHitOutputPort=off  CountDataType=Unsigned  CountWordLen=12  CountFracLen=0  CountSampTime=1
  HDL Counter5 : hdlsllib/Sources/HDL Counter  CountType=Count limited  CountInit=0  CountStep=1  CountMax=1  CountFromType=Initial value  CountFrom=0  CountResetPort=on  CountLoadPort=off  CountEnbPort=on  CountDirPort=off  CountHitOutputPort=off  CountDataType=Unsigned  CountWordLen=1  CountFracLen=0  CountSampTime=1
  Logical Operator : Logic  Operator=OR  AllPortsSameDT=off  OutDataTypeStr=boolean
  Logical Operator{1,3,7..8} (4 alike) : Logic  Operator=NOT  AllPortsSameDT=off  OutDataTypeStr=boolean
  Logical Operator{2,4..6} (4 alike) : Logic  AllPortsSameDT=off  OutDataTypeStr=boolean
  Mux : Mux  Inputs=2
  NR CRC Encoder : whdledac/NR CRC Encoder  CRCType=CRC16  EnableCRCMaskPort=off  SimulateUsing=Code generation
      settings: SourceProductBaseCode=LH
  NR LDPC Encoder2 : whdledac/NR LDPC Encoder
      settings: SourceProductBaseCode=LH
  Sample Control Bus Creator : whdlutilities/Sample Control Bus Creator
      settings: SourceProductBaseCode=LH
  Sample Control Bus Selector : whdlutilities/Sample Control Bus Selector  OutputSignals=start,end,valid
      settings: SourceProductBaseCode=LH
  Sample Control Bus Selector1 : whdlutilities/Sample Control Bus Selector  OutputSignals=start,end,valid
      settings: SourceProductBaseCode=LH
  Simple Dual Port RAM1 : hdlsllib/HDL RAMs/Simple Dual Port RAM  ram_size=12
      settings: SourceProductBaseCode=SL
  Subsystem : Subsystem
  Switch : Switch  Criteria=u2 ~= 0  SaturateOnIntegerOverflow=off  InputSameDT=off
  Switch1 : Switch  Criteria=u2 ~= 0  SaturateOnIntegerOverflow=off  InputSameDT=off
  Switch2 : Switch  Criteria=u2 ~= 0  SaturateOnIntegerOverflow=off  InputSameDT=off
  ctrl_gen : Subsystem
  valid_recover : Subsystem
  bit_level_process : Outport  OutDataTypeStr=boolean
  "bit_level_ctrl_process " : Outport  Port=2  OutDataTypeStr=Bus: samplecontrol
  wires:
  ctrl_gen/1(data_out) -> bit_level_process/1  "INTERLEAVE"
  process_valid/1 -> NR CRC Encoder/2
  Delay2/1 -> ctrl_gen/2(select_valid)
  Delay1/1 -> Mux/2
  Compare To Constant4/1 -> Logical Operator2/2
  Mux/1 -> ctrl_gen/1(data_in)
  Sample Control Bus Creator/1 -> NR LDPC Encoder2/2
  NR CRC Encoder/2 -> Sample Control Bus Selector/1
  Compare To Constant1/1 -> Logical Operator/1
  Compare To Constant2/1 -> HDL Counter5/2
  Constant2/1 -> Switch/3
  Compare To Constant6/1 -> Logical Operator6/2
  HDL Counter4/1 -> Compare To Constant2/1, Compare To Constant3/1, Compare To Constant4/1, Compare To Constant1/1  "wr_addr"
  Data Type Conversion1/1 -> Simple Dual Port RAM1/1  "wr_din"
  Compare To Constant5/1 -> Logical Operator6/1
  Logical Operator5/1 -> Simple Dual Port RAM1/3, Switch1/2, HDL Counter1/2  "wr_en"
  Compare To Constant3/1 -> Logical Operator/2
  Subsystem/1(end_out) -> valid_recover/3(end_in)
  process_data/1 -> NR CRC Encoder/1
  Data Type Conversion2/1 -> HDL Counter4/1
  Switch1/1 -> Simple Dual Port RAM1/2  "wr_addr"
  Logical Operator6/1 -> Switch/2, Delay2/1, Logical Operator7/1, Switch2/2, HDL Counter2/2
  Logical Operator1/1 -> HDL Counter1/1
  valid_recover/1(data_out) -> NR LDPC Encoder2/1
  NR LDPC Encoder2/2 -> Sample Control Bus Selector1/1
  HDL Counter1/1 -> Compare To Constant5/1, Compare To Constant6/1, Switch1/1
  Switch2/1 -> Simple Dual Port RAM1/4  "rd_addr"
  valid_recover/4(valid_out) -> Sample Control Bus Creator/3
  Logical Operator/1 -> Logical Operator2/1
  Logical Operator4/1 -> Logical Operator5/2
  Logical Operator3/1 -> Logical Operator4/1
  Logical Operator7/1 -> HDL Counter2/1
  Logical Operator2/1 -> Logical Operator5/1
  Sample Control Bus Selector1/3 -> Logical Operator4/2, Logical Operator1/1, Logical Operator8/1, HDL Counter4/2  "<valid>"
  valid_recover/3(end_out) -> Sample Control Bus Creator/2
  valid_recover/2(start_out) -> Sample Control Bus Creator/1
  Sample Control Bus Selector/1 -> valid_recover/2(start_in)  "<start>"
  Simple Dual Port RAM1/1 -> Data Type Conversion3/1
  NR LDPC Encoder2/1 -> Data Type Conversion1/1, Switch/1  "LDPC"
  Sample Control Bus Selector/2 -> Subsystem/1(end_in)  "<end>"
  Logical Operator8/1 -> HDL Counter5/1
  HDL Counter2/1 -> Switch2/1  "rd_addr"
  Constant1/1 -> NR LDPC Encoder2/4
  ctrl_gen/2(ctrl_out) -> "bit_level_ctrl_process "/1
  NR CRC Encoder/1 -> valid_recover/1(data_in)  "CRC"
  Constant3/1 -> Switch1/3, Switch2/3
  Constant/1 -> NR LDPC Encoder2/3
  Data Type Conversion3/1 -> Mux/1
  HDL Counter5/1 -> Data Type Conversion2/1, Logical Operator3/1  "loop_ctrl"
  Switch/1 -> Delay1/1

== system tx2/Subsystem1/mapping_process_L1 ==
  data_in : Inport  OutDataTypeStr=boolean
  mapping_ctrl : Inport  Port=2  OutDataTypeStr=Bus: samplecontrol
  Constant : Constant  Value=sqrt(2)/2  OutDataTypeStr=fixdt(1,16,14)
  Constant1 : Constant  Value=-sqrt(2)/2  OutDataTypeStr=fixdt(1,16,14)
  Constant2 : Constant  Value=0  OutDataTypeStr=uint8
  Constant3 : Constant  Value=0  OutDataTypeStr=fixdt(1,16,14)
  Delay : Delay  DelayLength=1  InitialCondition=0  ShowEnablePort=on
      settings: InputPortMap=u0,e6
  Delay{1,5..8,10..12} (8 alike) : Delay  DelayLength=1  InitialCondition=0
  Delay{3..4,9,13} (4 alike) : Delay  InitialCondition=0
  Delay2 : Delay  DelayLength=1  InitialCondition=0  ShowEnablePort=on
      settings: InputPortMap=u0,e6
  Demux : Demux  Outputs=2
  Logical Operator : Logic  Operator=OR  AllPortsSameDT=off  OutDataTypeStr=boolean
  Logical Operator1 : Logic  AllPortsSameDT=off  OutDataTypeStr=boolean
  Logical Operator13 : Logic  Operator=NOT  AllPortsSameDT=off  OutDataTypeStr=boolean
  Real-Imag to Complex : RealImagToComplex
  Real-Imag to Complex1 : RealImagToComplex
  Sample Control Bus Creator : whdlutilities/Sample Control Bus Creator
      settings: SourceProductBaseCode=LH
  Sample Control Bus Creator1 : whdlutilities/Sample Control Bus Creator
      settings: SourceProductBaseCode=LH
  Sample Control Bus Selector : whdlutilities/Sample Control Bus Selector  OutputSignals=start,end,valid
      settings: SourceProductBaseCode=LH
  Switch{,1..3} (4 alike) : Switch  Criteria=u2 ~= 0  SaturateOnIntegerOverflow=off  InputSameDT=off
  "divide6 " : hdlsllib/Sources/HDL Counter  CountType=Count limited  CountInit=1  CountStep=1  CountMax=12  CountFromType=Initial value  CountFrom=1  CountResetPort=on  CountLoadPort=off  CountEnbPort=on  CountDirPort=off  CountHitOutputPort=on  CountDataType=Unsigned  CountWordLen=8  CountFracLen=0  CountSampTime=1
  divide6 1 : hdlsllib/Sources/HDL Counter  CountType=Count limited  CountInit=1  CountStep=1  CountMax=6*12  CountFromType=Initial value  CountFrom=1  CountResetPort=on  CountLoadPort=off  CountEnbPort=on  CountDirPort=off  CountHitOutputPort=off  CountDataType=Unsigned  CountWordLen=8  CountFracLen=0  CountSampTime=1
  data_out : Outport  VectorParamsAs1DForOutWhenUnconnected=off
      settings: SignalType=complex
  ctrl_mapping : Outport  Port=2  OutDataTypeStr=Bus: samplecontrol  VectorParamsAs1DForOutWhenUnconnected=off
  RB_ctrl : Outport  Port=3  OutDataTypeStr=Bus: samplecontrol  VectorParamsAs1DForOutWhenUnconnected=off
  RB_id : Outport  Port=4  OutDataTypeStr=uint8  VectorParamsAs1DForOutWhenUnconnected=off
  wires:
  Constant1/1 -> Switch1/1, Switch/1
  Constant/1 -> Switch/3, Switch1/3
  Delay13/1 -> Switch3/2
  Real-Imag to Complex1/1 -> Switch3/3
  Constant3/1 -> Real-Imag to Complex1/1, Real-Imag to Complex1/2
  Switch3/1 -> data_out/1
  data_in/1 -> Delay/1  "data_with_CP"
  Sample Control Bus Creator1/1 -> RB_ctrl/1
  Delay7/1 -> RB_id/1
  Delay5/1 -> ctrl_mapping/1
  Delay12/1 -> Sample Control Bus Creator1/3
  Delay11/1 -> Sample Control Bus Creator1/2
  Delay8/1 -> Sample Control Bus Creator1/1
  Logical Operator1/1 -> Delay8/1
  Delay10/1 -> Logical Operator/1
  Delay9/1 -> Logical Operator/2
  Logical Operator/1 -> Logical Operator1/2
  Delay6/1 -> Switch3/1
  Constant2/1 -> Switch2/3
  Switch2/1 -> Delay7/1
  Delay4/1 -> Logical Operator1/1, Switch2/2, Delay12/1, "divide6 "/2, Logical Operator13/1
  divide6 1/1 -> Switch2/1  "RB_id"
  Sample Control Bus Creator/1 -> Delay3/1
  Sample Control Bus Selector/3 -> Delay/2, Delay1/1, Delay4/1, Sample Control Bus Creator/3  "<valid>"
  Sample Control Bus Selector/2 -> Sample Control Bus Creator/2  "<end>"
  Sample Control Bus Selector/1 -> Sample Control Bus Creator/1, Delay9/1  "<start>"
  Logical Operator13/1 -> "divide6 "/1, divide6 1/1
  "divide6 "/2 -> Delay10/1, Delay11/1, divide6 1/2  "count6"
  mapping_ctrl/1 -> Sample Control Bus Selector/1
  Delay1/1 -> Delay13/1, Delay2/2
  Delay3/1 -> Delay5/1
  Delay2/1 -> Delay6/1
  Real-Imag to Complex/1 -> Delay2/1
  Demux/2 -> Switch1/2
  Demux/1 -> Switch/2
  Delay/1 -> Demux/1
  Switch/1 -> Real-Imag to Complex/1
  Switch1/1 -> Real-Imag to Complex/2

== system tx2/Subsystem10/BF ==
  layer_data_in1 : Inport
  BF_data_ctrl : Inport  Port=2  OutDataTypeStr=Bus: samplecontrol
  RB_id : Inport  Port=3  OutDataTypeStr=uint8
  RB_id_ctrl : Inport  Port=4  OutDataTypeStr=Bus: samplecontrol
  Delay{,3..8,10} (8 alike) : Delay  DelayLength=1  InitialCondition=0
  Delay1 : Delay  InitialCondition=0
  Delay2 : Delay  DelayLength=3  InitialCondition=0
  Delay9 : Delay  InitialCondition=0
  Logical Operator : Logic  Operator=NOT  AllPortsSameDT=off  OutDataTypeStr=boolean
  Mux : Mux  Inputs=8
  Product{,1..7} (8 alike) : Product  OutDataTypeStr=fixdt(1,16,14)  LockScale=on
  Sample Control Bus Selector : whdlutilities/Sample Control Bus Selector  OutputSignals=start,end,valid
      settings: SourceProductBaseCode=LH
  Sample Control Bus Selector1 : whdlutilities/Sample Control Bus Selector  OutputSignals=start,end,valid
      settings: SourceProductBaseCode=LH
  address controller : hdlsllib/Sources/HDL Counter  CountType=Count limited  CountInit=0  CountStep=1  CountMax=7  CountFromType=Initial value  CountFrom=0  CountResetPort=on  CountLoadPort=off  CountEnbPort=on  CountDirPort=off  CountHitOutputPort=off  CountDataType=Unsigned  CountWordLen=8  CountFracLen=0  CountSampTime=1
  rom_bf1 : Subsystem
  rom_bf2 : Subsystem
  rom_bf3 : Subsystem
  rom_bf4 : Subsystem
  rom_bf5 : Subsystem
  rom_bf6 : Subsystem
  rom_bf7 : Subsystem
  rom_bf8 : Subsystem
  process_bf : Outport  PortDimensions=8  VectorParamsAs1DForOutWhenUnconnected=off
  BF_ctrl : Outport  Port=2  OutDataTypeStr=Bus: samplecontrol  VectorParamsAs1DForOutWhenUnconnected=off
  RB_n_bf : Outport  Port=3  VectorParamsAs1DForOutWhenUnconnected=off
  wires:
  Delay1/1 -> Product7/1, Product6/1, Product5/1, Product4/1, Product3/1, Product2/1, Product1/1, Product/1
  rom_bf1/1(data_out) -> Product/2
  Product/1 -> Delay/1
  Delay2/1 -> BF_ctrl/1  "BF_ctrl"
  address controller/1 -> rom_bf7/1(address), rom_bf8/1(address), rom_bf6/1(address), rom_bf5/1(address), rom_bf4/1(address), rom_bf3/1(address), rom_bf2/1(address), rom_bf1/1(address)
  Delay9/1 -> RB_n_bf/1  "RB_ID"
  RB_id_ctrl/1 -> Sample Control Bus Selector1/1
  BF_data_ctrl/1 -> Delay2/1, Sample Control Bus Selector/1
  Sample Control Bus Selector1/2 -> address controller/2  "<end>"
  RB_id/1 -> Delay9/1
  layer_data_in1/1 -> Delay1/1
  Sample Control Bus Selector/3 -> rom_bf2/2(read_en), rom_bf1/2(read_en), rom_bf3/2(read_en), rom_bf4/2(read_en), rom_bf5/2(read_en), rom_bf6/2(read_en), rom_bf7/2(read_en), rom_bf8/2(read_en)  "<valid>"
  Product1/1 -> Delay3/1
  Product2/1 -> Delay4/1
  Product4/1 -> Delay6/1
  Product3/1 -> Delay5/1
  Product5/1 -> Delay7/1
  Product6/1 -> Delay8/1
  rom_bf2/1(data_out) -> Product1/2
  rom_bf3/1(data_out) -> Product2/2
  rom_bf4/1(data_out) -> Product3/2
  rom_bf5/1(data_out) -> Product4/2
  rom_bf6/1(data_out) -> Product5/2
  Product7/1 -> Delay10/1
  rom_bf7/1(data_out) -> Product6/2
  rom_bf8/1(data_out) -> Product7/2
  Delay3/1 -> Mux/2
  Delay4/1 -> Mux/3
  Delay5/1 -> Mux/4
  Delay10/1 -> Mux/8
  Delay8/1 -> Mux/7
  Delay7/1 -> Mux/6
  Delay6/1 -> Mux/5
  Delay/1 -> Mux/1
  Mux/1 -> process_bf/1
  Sample Control Bus Selector1/3 -> Logical Operator/1  "<valid>"
  Logical Operator/1 -> address controller/1

== system tx2/Subsystem10/OFDM_process1 ==
  process_bf : Inport
  BF_ctrl : Inport  Port=2
  Demux : Demux  Outputs=8
  OFDM_process1_bf1 : Subsystem
  OFDM_process1_bf2 : Subsystem
  OFDM_process1_bf3 : Subsystem
  OFDM_process1_bf4 : Subsystem
  OFDM_process1_bf5 : Subsystem
  OFDM_process1_bf6 : Subsystem
  OFDM_process1_bf7 : Subsystem
  OFDM_process1_bf8 : Subsystem
  OFDM_bf1 : Outport
  OFDM_ctrl_bf1 : Outport  Port=2
  OFDM_bf2 : Outport  Port=3
  OFDM_ctrl_bf2 : Outport  Port=4
  OFDM_bf3 : Outport  Port=5
  OFDM_ctrl_bf3 : Outport  Port=6
  OFDM_bf4 : Outport  Port=7
  OFDM_ctrl_bf4 : Outport  Port=8
  OFDM_bf5 : Outport  Port=9
  OFDM_ctrl_bf5 : Outport  Port=10
  OFDM_bf6 : Outport  Port=11
  OFDM_ctrl_bf6 : Outport  Port=12
  OFDM_bf7 : Outport  Port=13
  OFDM_ctrl_bf7 : Outport  Port=14
  OFDM_bf8 : Outport  Port=15
  OFDM_ctrl_bf8 : Outport  Port=16
  wires:
  OFDM_process1_bf2/1(OFDM_process) -> OFDM_bf2/1
  OFDM_process1_bf4/1(OFDM_process) -> OFDM_bf4/1
  OFDM_process1_bf7/1(OFDM_process) -> OFDM_bf7/1
  process_bf/1 -> Demux/1
  OFDM_process1_bf5/2(OFDM_ctrl_process) -> OFDM_ctrl_bf5/1
  OFDM_process1_bf3/2(OFDM_ctrl_process) -> OFDM_ctrl_bf3/1
  OFDM_process1_bf4/2(OFDM_ctrl_process) -> OFDM_ctrl_bf4/1
  OFDM_process1_bf8/1(OFDM_process) -> OFDM_bf8/1
  OFDM_process1_bf1/1(OFDM_process) -> OFDM_bf1/1
  OFDM_process1_bf5/1(OFDM_process) -> OFDM_bf5/1
  OFDM_process1_bf6/2(OFDM_ctrl_process) -> OFDM_ctrl_bf6/1
  OFDM_process1_bf3/1(OFDM_process) -> OFDM_bf3/1
  OFDM_process1_bf6/1(OFDM_process) -> OFDM_bf6/1
  OFDM_process1_bf7/2(OFDM_ctrl_process) -> OFDM_ctrl_bf7/1
  Demux/6 -> OFDM_process1_bf6/1(data)  "bf6"
  Demux/7 -> OFDM_process1_bf7/1(data)  "bf7"
  Demux/8 -> OFDM_process1_bf8/1(data)  "bf8"
  OFDM_process1_bf8/2(OFDM_ctrl_process) -> OFDM_ctrl_bf8/1
  Demux/4 -> OFDM_process1_bf4/1(data)  "bf4"
  Demux/2 -> OFDM_process1_bf2/1(data)  "bf2"
  OFDM_process1_bf2/2(OFDM_ctrl_process) -> OFDM_ctrl_bf2/1
  OFDM_process1_bf1/2(OFDM_ctrl_process) -> OFDM_ctrl_bf1/1
  Demux/5 -> OFDM_process1_bf5/1(data)  "bf5"
  BF_ctrl/1 -> OFDM_process1_bf1/2(BF_ctrl), OFDM_process1_bf2/2(BF_ctrl), OFDM_process1_bf3/2(BF_ctrl), OFDM_process1_bf4/2(BF_ctrl), OFDM_process1_bf5/2(BF_ctrl), OFDM_process1_bf6/2(BF_ctrl), OFDM_process1_bf8/2(BF_ctrl), OFDM_process1_bf7/2(BF_ctrl)
  Demux/1 -> OFDM_process1_bf1/1(data)  "bf1"
  Demux/3 -> OFDM_process1_bf3/1(data)  "bf3"
